simulink model "towing_project"  (Simulink 10.1)
settings: Solver=ode4  StartTime=0.0  StopTime=1000  FixedStep=1  RelTol=1e-3  EnableMultiTasking=on
PreLoadFcn:
  | load('Initialization_data.mat');
values from neighbouring files (symbols this model uses):
  D1 = [MM(1,1)/100, 0, 0; 0, MM(2,2)/40, 0; 0, 0, MM(3,3)/20]    [initail_data.m]
  M1 = diag([6.25e5, 6.25e5, 6.25e5*7.5^2])    [initail_data.m]
  Ma1 = [7.58e4, 0, 0; 0, 3.69e5 -1.4e5; 0, -1.4e5, 8.77e6]    [initail_data.m]
  p00 = [0, 0, 0]'    [initail_data.m]
  p10 = [394, 237, 31]'    [initail_data.m]
  p20 = [394, -237, -31]'    [initail_data.m]
undefined symbols (not defined in the file or in its folder): D, M, Ma, magnitude
libraries: simulink x6, simulink_extras x2
settings Model: Creator=Lither  LastModifiedBy=Administrator
settings DataIOCC: LimitDataPoints=on
settings OptimizationCC: ExpressionDepthLimit=2147483647
settings DebuggingCC: FcnCallInpInsideContextMsg=warning  StateNameClashWarn=warning
settings ConfigComp: CovSFcnEnable=off

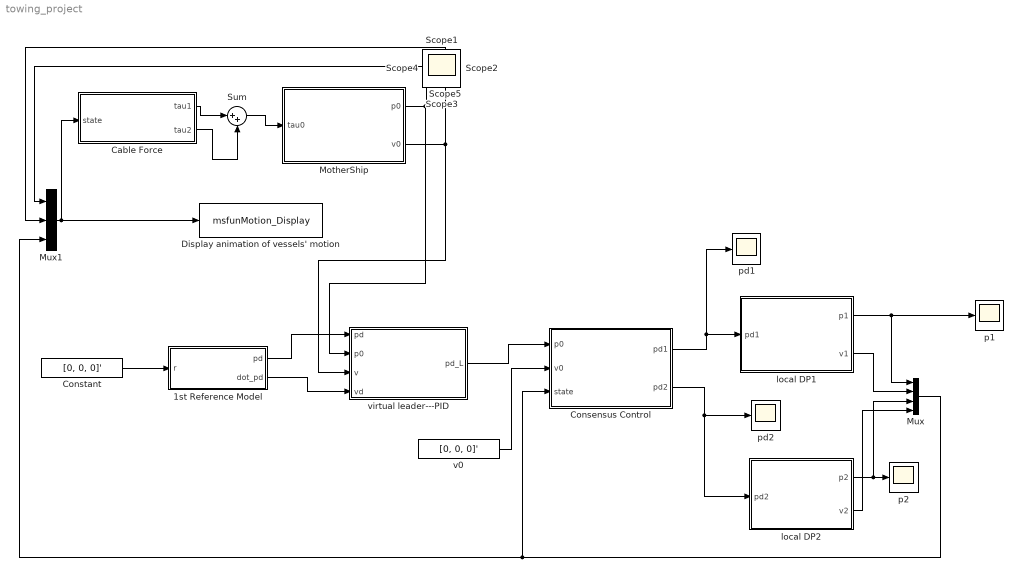
== system towing_project ==
  1st Reference Model : Subsystem  mask{T=200}
      mask prompts: T "Time constant of reference model"
  Cable Force : MATLAB Function  TreatAsAtomicUnit=on
  Consensus Control : MATLAB Function  TreatAsAtomicUnit=on
  Constant : Constant  Value=[0, 0, 0]'
  Display animation of vessels' motion : M-S-Function  FunctionName=msfunMotion_Display  Parameters=p00, p10, p20
  MotherShip : Subsystem  mask{wv=on}
      mask prompts: wv "Display animation of the vessel's motion"
  Mux : Mux
  Mux1 : Mux  Inputs=3
  Sum : Sum  Inputs=|++
  local DP1 : Subsystem
  local DP2 : Subsystem
  p1 : Scope
  p2 : Scope
  pd1 : Scope
  pd2 : Scope
  v0 : Constant  Value=[0, 0, 0]'
  virtual leader---PID : Subsystem  mask{Kp_L=diag([1, 1, 1]), Kd_L=diag([1, 1, 1])*0.1, Ki_L=diag([1, 1, 1])*0.01}
      mask prompts: Kp_L "比例增益：Kp_L"; Kd_L "微分增益：Kd_L"; Ki_L "积分增益：Ki_L"
  Scope{,1..5} (6 alike) : Scope
  wires:
  Consensus Control/1(pd1) -> pd1/1, local DP1/1(pd1)
  local DP1/1(p1) -> p1/1, Mux/1
  local DP1/2(v1) -> Mux/2
  local DP2/1(p2) -> Mux/3, p2/1
  local DP2/2(v2) -> Mux/4
  Mux/1 -> Consensus Control/3(state), Mux1/3
  Consensus Control/2(pd2) -> local DP2/1(pd2), pd2/1
  Mux1/1 -> Display animation of vessels' motion/1, Cable Force/1(state)
  Constant/1 -> 1st Reference Model/1(r)
  MotherShip/1(p0) -> virtual leader---PID/2(p0), Mux1/1
  MotherShip/2(v0) -> Mux1/2, virtual leader---PID/3(v)
  Sum/1 -> MotherShip/1(tau0)
  1st Reference Model/1(pd) -> virtual leader---PID/1(pd)
  1st Reference Model/2(dot_pd) -> virtual leader---PID/4(vd)
  virtual leader---PID/1(pd_L) -> Consensus Control/1(p0)
  v0/1 -> Consensus Control/2(v0)
  Cable Force/1(tau1) -> Sum/1
  Cable Force/2(tau2) -> Sum/2

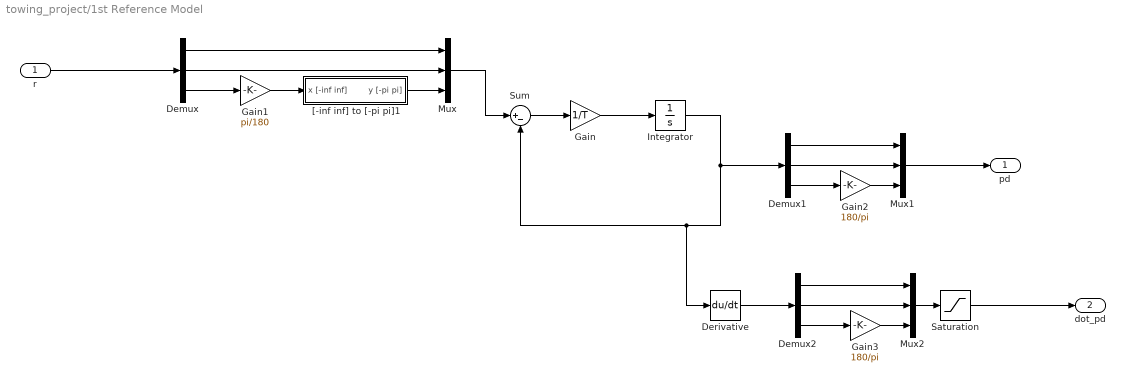
== system towing_project/1st Reference Model ==
  r : Inport
  Demux : Demux  Outputs=3
  Demux1 : Demux  Outputs=3
  Demux2 : Demux  Outputs=3
  Derivative : Derivative
  Gain : Gain  Gain=1/T
  Gain1 : Gain  Gain=pi/180
  Gain2 : Gain  Gain=180/pi
  Gain3 : Gain  Gain=180/pi
  Integrator : Integrator  InitialCondition=p00
  Mux : Mux  Inputs=3
  Mux1 : Mux  Inputs=3
  Mux2 : Mux  Inputs=3
  Saturation : Saturate  UpperLimit=10  LowerLimit=-10
  Sum : Sum  Inputs=|+-
  "[-inf inf] to [-pi pi]1" : Subsystem
  pd : Outport
  dot_pd : Outport  Port=2
  wires:
  Integrator/1 -> Derivative/1, Sum/2, Demux1/1
  Sum/1 -> Gain/1
  Gain/1 -> Integrator/1
  Saturation/1 -> dot_pd/1
  r/1 -> Demux/1
  Demux/3 -> Gain1/1
  Demux/2 -> Mux/2
  Demux/1 -> Mux/1
  Mux/1 -> Sum/1
  Demux1/3 -> Gain2/1
  Gain2/1 -> Mux1/3
  Demux1/2 -> Mux1/2
  Demux1/1 -> Mux1/1
  Mux1/1 -> pd/1
  Demux2/3 -> Gain3/1
  Demux2/2 -> Mux2/2
  Demux2/1 -> Mux2/1
  Gain3/1 -> Mux2/3
  Derivative/1 -> Demux2/1
  Mux2/1 -> Saturation/1
  Gain1/1 -> "[-inf inf] to [-pi pi]1"/1(x [-inf inf])
  "[-inf inf] to [-pi pi]1"/1(y [-pi pi]) -> Mux/3

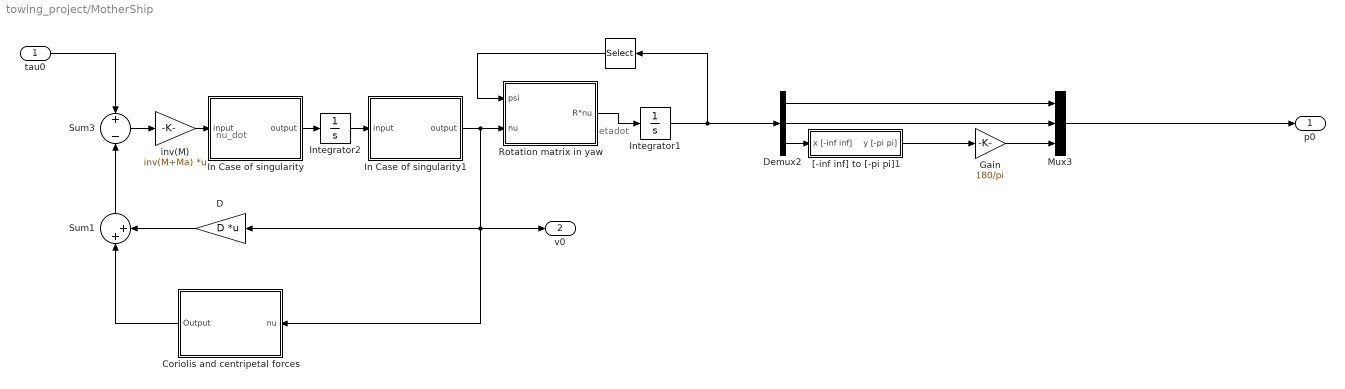
== system towing_project/MotherShip ==
  note: nu_dot
  note: etadot
  tau0 : Inport
  " " : Selector  InputPortWidth=3  IndexOptions=Index vector (dialog)  Indices=[3]  OutputSizes=1
  Coriolis and centripetal forces : Subsystem
  D : Gain  Gain=D  Multiplication=Matrix(K*u)  SaturateOnIntegerOverflow=on  OutDataTypeStr=Inherit: Same as input  ParamDataTypeStr=Inherit: Same as input
  Demux2 : Demux  Outputs=3
  Gain : Gain  Gain=180/pi
  In Case of singularity : Subsystem
  In Case of singularity1 : Subsystem
  Integrator1 : Integrator  InitialCondition=[p00(1), p00(2), p00(3)/180*pi]'
  Integrator2 : Integrator
  Mux3 : Mux  Inputs=3
  Rotation matrix in yaw : Subsystem
  Sum1 : Sum  Inputs=|++  InputSameDT=on  SaturateOnIntegerOverflow=on  OutDataTypeStr=Inherit: Same as first input
  Sum3 : Sum  Inputs=+-  InputSameDT=on  SaturateOnIntegerOverflow=on  OutDataTypeStr=Inherit: Same as first input
  "[-inf inf] to [-pi pi]1" : Subsystem
  inv(M) : Gain  Gain=inv(M+Ma)  Multiplication=Matrix(K*u)  SaturateOnIntegerOverflow=on  OutDataTypeStr=Inherit: Same as input  ParamDataTypeStr=Inherit: Same as input
  p0 : Outport
  v0 : Outport  Port=2
  wires:
  Sum3/1 -> inv(M)/1
  inv(M)/1 -> In Case of singularity/1(input)
  Rotation matrix in yaw/1(R*nu) -> Integrator1/1
  Integrator1/1 -> Demux2/1, " "/1
  " "/1 -> Rotation matrix in yaw/1(psi)
  tau0/1 -> Sum3/1
  Integrator2/1 -> In Case of singularity1/1(input)
  In Case of singularity/1(output) -> Integrator2/1
  In Case of singularity1/1(output) -> Rotation matrix in yaw/2(nu), D/1, Coriolis and centripetal forces/1(nu), v0/1
  D/1 -> Sum1/2
  Coriolis and centripetal forces/1(Output) -> Sum1/1
  Sum1/1 -> Sum3/2
  Demux2/3 -> "[-inf inf] to [-pi pi]1"/1(x [-inf inf])
  Demux2/1 -> Mux3/1
  Demux2/2 -> Mux3/2
  Mux3/1 -> p0/1
  "[-inf inf] to [-pi pi]1"/1(y [-pi pi]) -> Gain/1
  Gain/1 -> Mux3/3

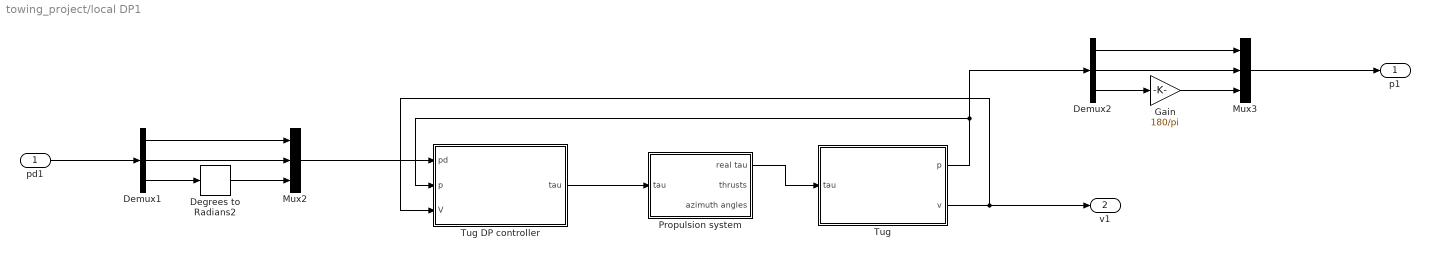
== system towing_project/local DP1 ==
  pd1 : Inport
  Degrees to Radians2 : simulink_extras/Transformations/Degrees to Radians
  Demux1 : Demux  Outputs=3
  Demux2 : Demux  Outputs=3
  Gain : Gain  Gain=180/pi
  Mux2 : Mux  Inputs=3
  Mux3 : Mux  Inputs=3
  Propulsion system : Subsystem  mask{f0=[1;1;1], a0=[50;60;70], u0=[1; 1; 1], wa=on}
      mask prompts: f0 "Initial values of thrusts"; a0 "Initial values of azimuth angles"; u0 "Thruster utilization"; wa "Show animation of thrust and azimuth angle"
  Tug : Subsystem  mask{wv=on}
      mask prompts: wv "Display animation of the vessel's motion"
  Tug DP controller : Subsystem  mask(Nonlinear DP Controller){Kp=diag([0.0028, 0.004, 0.0031]), Kd=diag([0.0573, 0.0716, 0.025]), Ki=diag([0.0028, 0.004, 0.0031])*0.01, WFF_gain=0}
      mask prompts: Kp "Proportional Gain Matrix: Kp"; Kd "Derivative Gain Matrix: Kd"; Ki "Integral Gain Matrix: Ki"; WFF_gain "Wave feedforward Gain"
      mask help: PID controller for Set-Point Reulation in Surge, Sway and Yaw
      mask Help:
      | The nonlinear  PID controller uses the rotation matrix in yaw for proper scaling of the surge, sway and yaw gains as a function of the yaw angle.
      | INPUTS: (1) eta_ref, (2) eta, (3) nu. OUPUTS: (1) tau.
      mask Display: disp('PID controller')
  p1 : Outport
  v1 : Outport  Port=2
  wires:
  Tug/2(v) -> v1/1, Tug DP controller/3(V)
  Tug DP controller/1(tau) -> Propulsion system/1(tau)
  Demux1/2 -> Mux2/2
  Mux2/1 -> Tug DP controller/1(pd)
  Demux1/1 -> Mux2/1
  Degrees to Radians2/1 -> Mux2/3
  Demux1/3 -> Degrees to Radians2/1
  pd1/1 -> Demux1/1
  Propulsion system/1(real tau) -> Tug/1(tau)
  Demux2/2 -> Mux3/2
  Tug/1(p) -> Demux2/1, Tug DP controller/2(p)
  Mux3/1 -> p1/1
  Demux2/3 -> Gain/1
  Gain/1 -> Mux3/3
  Demux2/1 -> Mux3/1

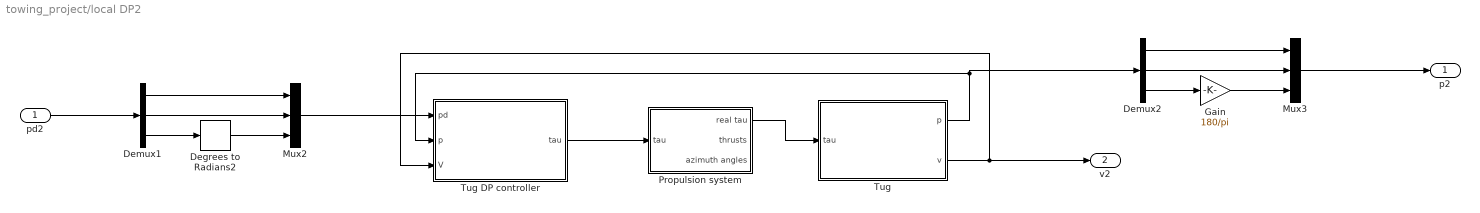
== system towing_project/local DP2 ==
  pd2 : Inport
  Degrees to Radians2 : simulink_extras/Transformations/Degrees to Radians
  Demux1 : Demux  Outputs=3
  Demux2 : Demux  Outputs=3
  Gain : Gain  Gain=180/pi
  Mux2 : Mux  Inputs=3
  Mux3 : Mux  Inputs=3
  Propulsion system : Subsystem  mask{f0=[1;1;1], a0=[50;60;70], u0=[1; 1; 1], wa=on}
      mask prompts: f0 "Initial values of thrusts"; a0 "Initial values of azimuth angles"; u0 "Thruster utilization"; wa "Show animation of thrust and azimuth angle"
  Tug : Subsystem  mask{wv=on}
      mask prompts: wv "Display animation of the vessel's motion"
  Tug DP controller : Subsystem  mask(Nonlinear DP Controller){Kp=diag([0.0028, 0.004, 0.0031]), Kd=diag([0.0573, 0.0716, 0.025]), Ki=diag([0.0028, 0.004, 0.0031])*0.01, WFF_gain=0}
      mask prompts: Kp "Proportional Gain Matrix: Kp"; Kd "Derivative Gain Matrix: Kd"; Ki "Integral Gain Matrix: Ki"; WFF_gain "Wave feedforward Gain"
      mask help: PID controller for Set-Point Reulation in Surge, Sway and Yaw
      mask Help:
      | The nonlinear  PID controller uses the rotation matrix in yaw for proper scaling of the surge, sway and yaw gains as a function of the yaw angle.
      | INPUTS: (1) eta_ref, (2) eta, (3) nu. OUPUTS: (1) tau.
      mask Display: disp('PID controller')
  p2 : Outport
  v2 : Outport  Port=2
  wires:
  Tug/2(v) -> v2/1, Tug DP controller/3(V)
  Tug DP controller/1(tau) -> Propulsion system/1(tau)
  Demux1/2 -> Mux2/2
  Mux2/1 -> Tug DP controller/1(pd)
  Demux1/1 -> Mux2/1
  Degrees to Radians2/1 -> Mux2/3
  Demux1/3 -> Degrees to Radians2/1
  pd2/1 -> Demux1/1
  Propulsion system/1(real tau) -> Tug/1(tau)
  Mux3/1 -> p2/1
  Tug/1(p) -> Demux2/1, Tug DP controller/2(p)
  Demux2/3 -> Gain/1
  Demux2/2 -> Mux3/2
  Gain/1 -> Mux3/3
  Demux2/1 -> Mux3/1

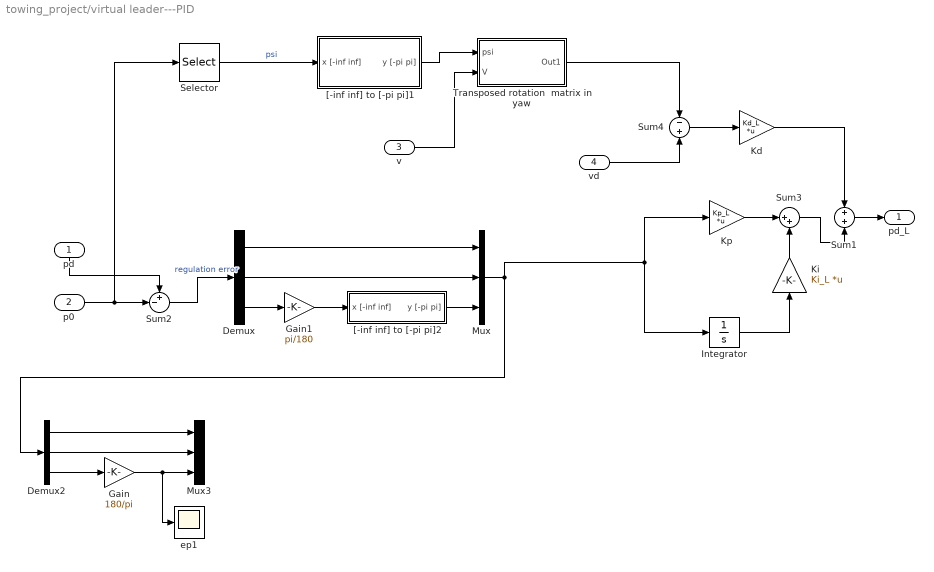
== system towing_project/virtual leader---PID ==
  pd : Inport
  p0 : Inport  Port=2
  v : Inport  Port=3
  vd : Inport  Port=4
  Demux : Demux  Outputs=3
  Demux2 : Demux  Outputs=3
  Gain : Gain  Gain=180/pi
  Gain1 : Gain  Gain=pi/180
  Integrator : Integrator
  Kd : Gain  Gain=Kd_L  Multiplication=Matrix(K*u)  SaturateOnIntegerOverflow=on  OutDataTypeStr=Inherit: Same as input  ParamDataTypeStr=Inherit: Same as input
  Ki : Gain  Gain=Ki_L  Multiplication=Matrix(K*u)  SaturateOnIntegerOverflow=on  OutDataTypeStr=Inherit: Same as input  ParamDataTypeStr=Inherit: Same as input
  Kp : Gain  Gain=Kp_L  Multiplication=Matrix(K*u)  SaturateOnIntegerOverflow=on  OutDataTypeStr=Inherit: Same as input  ParamDataTypeStr=Inherit: Same as input
  Mux : Mux  Inputs=3
  Mux3 : Mux  Inputs=3
  Selector : Selector  InputPortWidth=3  IndexOptions=Index vector (dialog)  Indices=[ 3]  OutputSizes=1
  Sum1 : Sum  InputSameDT=on  SaturateOnIntegerOverflow=on  OutDataTypeStr=Inherit: Same as first input
  Sum2 : Sum  Inputs=+-|  InputSameDT=on  SaturateOnIntegerOverflow=on  OutDataTypeStr=Inherit: Same as first input
  Sum3 : Sum  Inputs=|++  InputSameDT=on  SaturateOnIntegerOverflow=on  OutDataTypeStr=Inherit: Same as first input
  Sum4 : Sum  Inputs=-+  InputSameDT=on  SaturateOnIntegerOverflow=on  OutDataTypeStr=Inherit: Same as first input
  Transposed rotation  matrix in yaw : Subsystem
  "[-inf inf] to [-pi pi]1" : Subsystem
  "[-inf inf] to [-pi pi]2" : Subsystem
  ep1 : Scope
  pd_L : Outport  InitialOutput=0
  wires:
  Gain/1 -> ep1/1, Mux3/3
  Demux2/1 -> Mux3/1
  Kp/1 -> Sum3/1
  "[-inf inf] to [-pi pi]1"/1(y [-pi pi]) -> Transposed rotation  matrix in yaw/1(psi)
  Demux2/3 -> Gain/1
  Demux2/2 -> Mux3/2
  Integrator/1 -> Ki/1
  Sum1/1 -> pd_L/1
  p0/1 -> Sum2/2, Selector/1
  Sum2/1 -> Demux/1  "regulation error"
  pd/1 -> Sum2/1
  Mux/1 -> Demux2/1, Kp/1, Integrator/1
  Demux/1 -> Mux/1
  Selector/1 -> "[-inf inf] to [-pi pi]1"/1(x [-inf inf])  "psi"
  Ki/1 -> Sum3/2
  Demux/2 -> Mux/2
  "[-inf inf] to [-pi pi]2"/1(y [-pi pi]) -> Mux/3
  Demux/3 -> Gain1/1
  Gain1/1 -> "[-inf inf] to [-pi pi]2"/1(x [-inf inf])
  v/1 -> Transposed rotation  matrix in yaw/2(V)
  Sum4/1 -> Kd/1
  Kd/1 -> Sum1/1
  Sum3/1 -> Sum1/2
  Transposed rotation  matrix in yaw/1(Out1) -> Sum4/1
  vd/1 -> Sum4/2

== system towing_project/1st Reference Model/[-inf inf] to [-pi pi]1 ==
  note: x
  note: r
  x [-inf inf] : Inport
  Constant : Constant  Value=2*pi
  Gain : Gain  Gain=pi  SaturateOnIntegerOverflow=on  OutDataTypeStr=Inherit: Same as input  ParamDataTypeStr=Inherit: Same as input
  Math Function : Math  Operator=rem  SignedPower=on  SaturateOnIntegerOverflow=on
  Saturation : Saturate  UpperLimit=1e10  LowerLimit=-1e10
  Sign : Signum
  Sum : Sum  Inputs=|+-  SaturateOnIntegerOverflow=on
  Sum1 : Sum  Inputs=|++  SaturateOnIntegerOverflow=on
  y [-pi pi] : Outport
  wires:
  x [-inf inf]/1 -> Saturation/1
  Sign/1 -> Gain/1
  Gain/1 -> Sum/2, Sum1/2
  Sum1/1 -> Math Function/1
  Constant/1 -> Math Function/2
  Math Function/1 -> Sum/1
  Sum/1 -> y [-pi pi]/1
  Saturation/1 -> Sum1/1, Sign/1

== system towing_project/MotherShip/Coriolis and centripetal forces ==
  nu : Inport
  Mux : Mux  Inputs=3
  Selector1 : Selector  InputPortWidth=3  IndexOptions=Index vector (dialog)  Indices=[1 ]  OutputSizes=1
  Selector2 : Selector  InputPortWidth=3  IndexOptions=Index vector (dialog)  Indices=[2]  OutputSizes=1
  Selector3 : Selector  InputPortWidth=3  IndexOptions=Index vector (dialog)  Indices=[3]  OutputSizes=1
  Subsystem : Subsystem
  Subsystem1 : Subsystem
  Subsystem2 : Subsystem
  Output : Outport
  wires:
  nu/1 -> Selector1/1, Selector2/1, Selector3/1
  Selector2/1 -> Subsystem/1(v), Subsystem2/2(v)  "v"
  Selector3/1 -> Subsystem/2(r), Subsystem1/2(r), Subsystem2/3(r)  "r"
  Selector1/1 -> Subsystem1/1(u), Subsystem2/1(u)  "u"
  Subsystem/1(x direction) -> Mux/1
  Subsystem1/1(y direction) -> Mux/2
  Subsystem2/1(yaw direction) -> Mux/3
  Mux/1 -> Output/1

== system towing_project/MotherShip/In Case of singularity ==
  input : Inport
  Compare To Constant : simulink/Logic and Bit Operations/Compare To Constant  relop=>=  const=1e8  OutDataTypeStr=boolean
  Stop Simulation : Stop
  output : Outport
  wires:
  input/1 -> output/1, Compare To Constant/1
  Compare To Constant/1 -> Stop Simulation/1

== system towing_project/MotherShip/In Case of singularity1 ==
  input : Inport
  Compare To Constant : simulink/Logic and Bit Operations/Compare To Constant  relop=>=  const=1e10  OutDataTypeStr=boolean
  Stop Simulation : Stop
  output : Outport
  wires:
  input/1 -> output/1, Compare To Constant/1
  Compare To Constant/1 -> Stop Simulation/1

== system towing_project/MotherShip/Rotation matrix in yaw ==
  psi : Inport
  nu : Inport  Port=2
  Fcn : Fcn  Expr=cos(u(1))*u(2)-sin(u(1))*u(3)
  Fcn1 : Fcn  Expr=sin(u(1))*u(2)+cos(u(1))*u(3)
  Fcn2 : Fcn  Expr=u(4)
  Mux : Mux  Inputs=2
  Mux1 : Mux  Inputs=3
  R*nu : Outport
  wires:
  Mux1/1 -> R*nu/1  "eta_dot"
  Mux/1 -> Fcn/1, Fcn1/1, Fcn2/1
  psi/1 -> Mux/1
  nu/1 -> Mux/2
  Fcn1/1 -> Mux1/2  "y_dot"
  Fcn/1 -> Mux1/1  "x_dot"
  Fcn2/1 -> Mux1/3  "psi_dot"

== system towing_project/MotherShip/[-inf inf] to [-pi pi]1 ==
  note: x
  note: r
  x [-inf inf] : Inport
  Constant : Constant  Value=2*pi
  Gain : Gain  Gain=pi  SaturateOnIntegerOverflow=on  OutDataTypeStr=Inherit: Same as input  ParamDataTypeStr=Inherit: Same as input
  Math Function : Math  Operator=rem  SignedPower=on  SaturateOnIntegerOverflow=on
  Saturation : Saturate  UpperLimit=1e10  LowerLimit=-1e10
  Sign : Signum
  Sum : Sum  Inputs=|+-  SaturateOnIntegerOverflow=on
  Sum1 : Sum  Inputs=|++  SaturateOnIntegerOverflow=on
  y [-pi pi] : Outport
  wires:
  x [-inf inf]/1 -> Saturation/1
  Sign/1 -> Gain/1
  Gain/1 -> Sum/2, Sum1/2
  Sum1/1 -> Math Function/1
  Constant/1 -> Math Function/2
  Math Function/1 -> Sum/1
  Sum/1 -> y [-pi pi]/1
  Saturation/1 -> Sum1/1, Sign/1

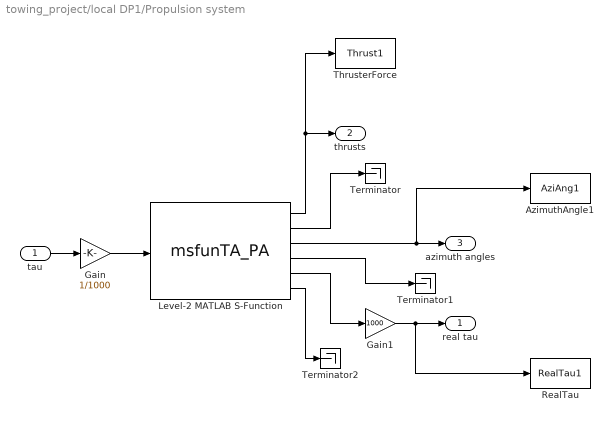
== system towing_project/local DP1/Propulsion system ==
  tau : Inport
  AzimuthAngle1 : ToWorkspace  VariableName=AziAng1  SampleTime=-1
  Gain : Gain  Gain=1/1000
  Gain1 : Gain  Gain=1000
  Level-2 MATLAB S-Function : M-S-Function  FunctionName=msfunTA_PA  Parameters=f0,a0,wa
  RealTau : ToWorkspace  VariableName=RealTau1  SampleTime=-1
  Terminator : Terminator
  Terminator1 : Terminator
  Terminator2 : Terminator
  ThrusterForce : ToWorkspace  VariableName=Thrust1  SampleTime=-1
  real tau : Outport
  thrusts : Outport  Port=2
  azimuth angles : Outport  Port=3
  wires:
  tau/1 -> Gain/1
  Level-2 MATLAB S-Function/2 -> Terminator/1
  Level-2 MATLAB S-Function/3 -> AzimuthAngle1/1, azimuth angles/1
  Level-2 MATLAB S-Function/4 -> Terminator1/1
  Level-2 MATLAB S-Function/5 -> Gain1/1
  Level-2 MATLAB S-Function/6 -> Terminator2/1
  Level-2 MATLAB S-Function/1 -> ThrusterForce/1, thrusts/1
  Gain/1 -> Level-2 MATLAB S-Function/1
  Gain1/1 -> RealTau/1, real tau/1

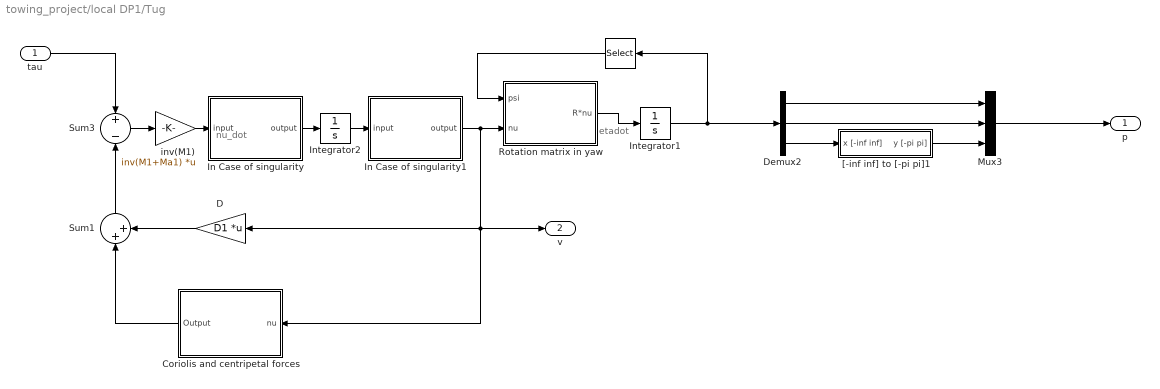
== system towing_project/local DP1/Tug ==
  note: nu_dot
  note: etadot
  tau : Inport
  " " : Selector  InputPortWidth=3  IndexOptions=Index vector (dialog)  Indices=[3]  OutputSizes=1
  Coriolis and centripetal forces : Subsystem
  D : Gain  Gain=D1  Multiplication=Matrix(K*u)  SaturateOnIntegerOverflow=on  OutDataTypeStr=Inherit: Same as input  ParamDataTypeStr=Inherit: Same as input
  Demux2 : Demux  Outputs=3
  In Case of singularity : Subsystem
  In Case of singularity1 : Subsystem
  Integrator1 : Integrator  InitialCondition=[p10(1), p10(2), p10(3)/180*pi]'
  Integrator2 : Integrator
  Mux3 : Mux  Inputs=3
  Rotation matrix in yaw : Subsystem
  Sum1 : Sum  Inputs=|++  InputSameDT=on  SaturateOnIntegerOverflow=on  OutDataTypeStr=Inherit: Same as first input
  Sum3 : Sum  Inputs=+-  InputSameDT=on  SaturateOnIntegerOverflow=on  OutDataTypeStr=Inherit: Same as first input
  "[-inf inf] to [-pi pi]1" : Subsystem
  inv(M1) : Gain  Gain=inv(M1+Ma1)  Multiplication=Matrix(K*u)  SaturateOnIntegerOverflow=on  OutDataTypeStr=Inherit: Same as input  ParamDataTypeStr=Inherit: Same as input
  p : Outport
  v : Outport  Port=2
  wires:
  Sum3/1 -> inv(M1)/1
  inv(M1)/1 -> In Case of singularity/1(input)
  Rotation matrix in yaw/1(R*nu) -> Integrator1/1
  Integrator1/1 -> Demux2/1, " "/1
  " "/1 -> Rotation matrix in yaw/1(psi)
  tau/1 -> Sum3/1
  Integrator2/1 -> In Case of singularity1/1(input)
  In Case of singularity/1(output) -> Integrator2/1
  In Case of singularity1/1(output) -> Rotation matrix in yaw/2(nu), D/1, Coriolis and centripetal forces/1(nu), v/1
  D/1 -> Sum1/2
  Coriolis and centripetal forces/1(Output) -> Sum1/1
  Sum1/1 -> Sum3/2
  Demux2/3 -> "[-inf inf] to [-pi pi]1"/1(x [-inf inf])
  Demux2/1 -> Mux3/1
  Demux2/2 -> Mux3/2
  "[-inf inf] to [-pi pi]1"/1(y [-pi pi]) -> Mux3/3
  Mux3/1 -> p/1

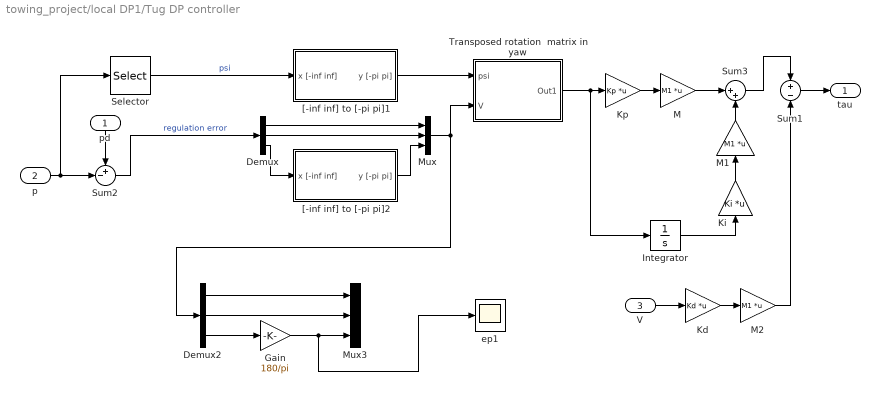
== system towing_project/local DP1/Tug DP controller ==
  pd : Inport
  p : Inport  Port=2
  V : Inport  Port=3
  Demux : Demux  Outputs=3
  Demux2 : Demux  Outputs=3
  Gain : Gain  Gain=180/pi
  Integrator : Integrator
  Kd : Gain  Gain=Kd  Multiplication=Matrix(K*u)  SaturateOnIntegerOverflow=on  OutDataTypeStr=Inherit: Same as input  ParamDataTypeStr=Inherit: Same as input
  Ki : Gain  Gain=Ki  Multiplication=Matrix(K*u)  SaturateOnIntegerOverflow=on  OutDataTypeStr=Inherit: Same as input  ParamDataTypeStr=Inherit: Same as input
  Kp : Gain  Gain=Kp  Multiplication=Matrix(K*u)  SaturateOnIntegerOverflow=on  OutDataTypeStr=Inherit: Same as input  ParamDataTypeStr=Inherit: Same as input
  M : Gain  Gain=M1  Multiplication=Matrix(K*u)  SaturateOnIntegerOverflow=on  OutDataTypeStr=Inherit: Same as input  ParamDataTypeStr=Inherit: Same as input
  M1 : Gain  Gain=M1  Multiplication=Matrix(K*u)  SaturateOnIntegerOverflow=on  OutDataTypeStr=Inherit: Same as input  ParamDataTypeStr=Inherit: Same as input
  M2 : Gain  Gain=M1  Multiplication=Matrix(K*u)  SaturateOnIntegerOverflow=on  OutDataTypeStr=Inherit: Same as input  ParamDataTypeStr=Inherit: Same as input
  Mux : Mux  Inputs=3
  Mux3 : Mux  Inputs=3
  Selector : Selector  InputPortWidth=3  IndexOptions=Index vector (dialog)  Indices=[ 3]  OutputSizes=1
  Sum1 : Sum  Inputs=+-  InputSameDT=on  SaturateOnIntegerOverflow=on  OutDataTypeStr=Inherit: Same as first input
  Sum2 : Sum  Inputs=+-|  InputSameDT=on  SaturateOnIntegerOverflow=on  OutDataTypeStr=Inherit: Same as first input
  Sum3 : Sum  Inputs=|++  InputSameDT=on  SaturateOnIntegerOverflow=on  OutDataTypeStr=Inherit: Same as first input
  Transposed rotation  matrix in yaw : Subsystem
  "[-inf inf] to [-pi pi]1" : Subsystem
  "[-inf inf] to [-pi pi]2" : Subsystem
  ep1 : Scope
  tau : Outport  InitialOutput=0
  wires:
  "[-inf inf] to [-pi pi]1"/1(y [-pi pi]) -> Transposed rotation  matrix in yaw/1(psi)
  Selector/1 -> "[-inf inf] to [-pi pi]1"/1(x [-inf inf])  "psi"
  Mux/1 -> Demux2/1, Transposed rotation  matrix in yaw/2(V)
  Demux/1 -> Mux/1
  Demux/2 -> Mux/2
  "[-inf inf] to [-pi pi]2"/1(y [-pi pi]) -> Mux/3
  Sum2/1 -> Demux/1  "regulation error"
  Demux/3 -> "[-inf inf] to [-pi pi]2"/1(x [-inf inf])
  pd/1 -> Sum2/1
  Sum1/1 -> tau/1
  p/1 -> Sum2/2, Selector/1
  V/1 -> Kd/1
  Integrator/1 -> Ki/1
  Kp/1 -> M/1
  Ki/1 -> M1/1
  Transposed rotation  matrix in yaw/1(Out1) -> Kp/1, Integrator/1
  Kd/1 -> M2/1
  M/1 -> Sum3/1
  M1/1 -> Sum3/2
  Sum3/1 -> Sum1/1
  M2/1 -> Sum1/2
  Demux2/3 -> Gain/1
  Demux2/1 -> Mux3/1
  Demux2/2 -> Mux3/2
  Gain/1 -> ep1/1, Mux3/3

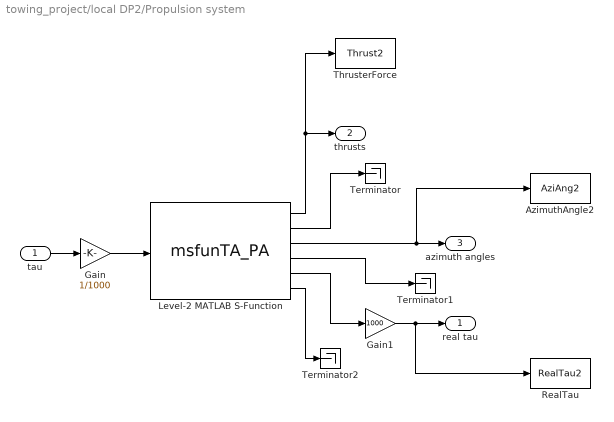
== system towing_project/local DP2/Propulsion system ==
  tau : Inport
  AzimuthAngle2 : ToWorkspace  VariableName=AziAng2  SampleTime=-1
  Gain : Gain  Gain=1/1000
  Gain1 : Gain  Gain=1000
  Level-2 MATLAB S-Function : M-S-Function  FunctionName=msfunTA_PA  Parameters=f0,a0,wa
  RealTau : ToWorkspace  VariableName=RealTau2  SampleTime=-1
  Terminator : Terminator
  Terminator1 : Terminator
  Terminator2 : Terminator
  ThrusterForce : ToWorkspace  VariableName=Thrust2  SampleTime=-1
  real tau : Outport
  thrusts : Outport  Port=2
  azimuth angles : Outport  Port=3
  wires:
  tau/1 -> Gain/1
  Level-2 MATLAB S-Function/2 -> Terminator/1
  Level-2 MATLAB S-Function/3 -> AzimuthAngle2/1, azimuth angles/1
  Level-2 MATLAB S-Function/4 -> Terminator1/1
  Level-2 MATLAB S-Function/5 -> Gain1/1
  Level-2 MATLAB S-Function/6 -> Terminator2/1
  Level-2 MATLAB S-Function/1 -> ThrusterForce/1, thrusts/1
  Gain/1 -> Level-2 MATLAB S-Function/1
  Gain1/1 -> RealTau/1, real tau/1

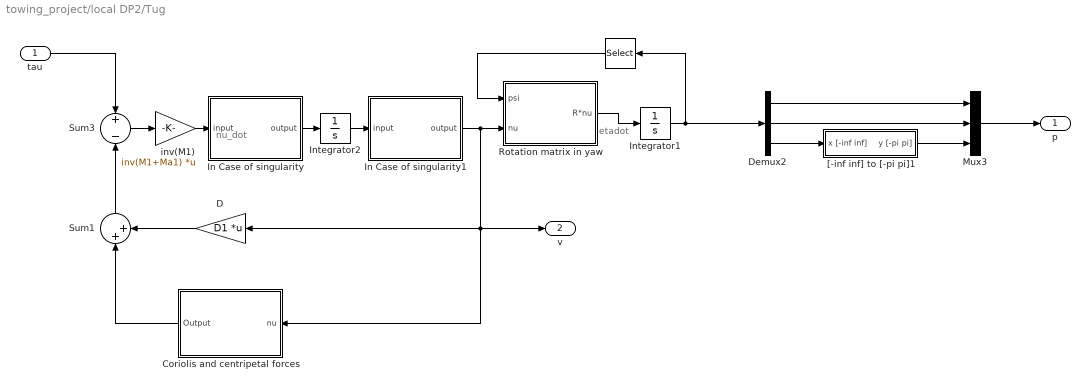
== system towing_project/local DP2/Tug ==
  note: nu_dot
  note: etadot
  tau : Inport
  " " : Selector  InputPortWidth=3  IndexOptions=Index vector (dialog)  Indices=[3]  OutputSizes=1
  Coriolis and centripetal forces : Subsystem
  D : Gain  Gain=D1  Multiplication=Matrix(K*u)  SaturateOnIntegerOverflow=on  OutDataTypeStr=Inherit: Same as input  ParamDataTypeStr=Inherit: Same as input
  Demux2 : Demux  Outputs=3
  In Case of singularity : Subsystem
  In Case of singularity1 : Subsystem
  Integrator1 : Integrator  InitialCondition=[p20(1), p20(2), p20(3)/180*pi]'
  Integrator2 : Integrator
  Mux3 : Mux  Inputs=3
  Rotation matrix in yaw : Subsystem
  Sum1 : Sum  Inputs=|++  InputSameDT=on  SaturateOnIntegerOverflow=on  OutDataTypeStr=Inherit: Same as first input
  Sum3 : Sum  Inputs=+-  InputSameDT=on  SaturateOnIntegerOverflow=on  OutDataTypeStr=Inherit: Same as first input
  "[-inf inf] to [-pi pi]1" : Subsystem
  inv(M1) : Gain  Gain=inv(M1+Ma1)  Multiplication=Matrix(K*u)  SaturateOnIntegerOverflow=on  OutDataTypeStr=Inherit: Same as input  ParamDataTypeStr=Inherit: Same as input
  p : Outport
  v : Outport  Port=2
  wires:
  Sum3/1 -> inv(M1)/1
  inv(M1)/1 -> In Case of singularity/1(input)
  Rotation matrix in yaw/1(R*nu) -> Integrator1/1
  " "/1 -> Rotation matrix in yaw/1(psi)
  tau/1 -> Sum3/1
  Integrator2/1 -> In Case of singularity1/1(input)
  In Case of singularity/1(output) -> Integrator2/1
  In Case of singularity1/1(output) -> Rotation matrix in yaw/2(nu), D/1, Coriolis and centripetal forces/1(nu), v/1
  D/1 -> Sum1/2
  Coriolis and centripetal forces/1(Output) -> Sum1/1
  Sum1/1 -> Sum3/2
  Demux2/3 -> "[-inf inf] to [-pi pi]1"/1(x [-inf inf])
  Integrator1/1 -> " "/1, Demux2/1
  "[-inf inf] to [-pi pi]1"/1(y [-pi pi]) -> Mux3/3
  Demux2/2 -> Mux3/2
  Demux2/1 -> Mux3/1
  Mux3/1 -> p/1

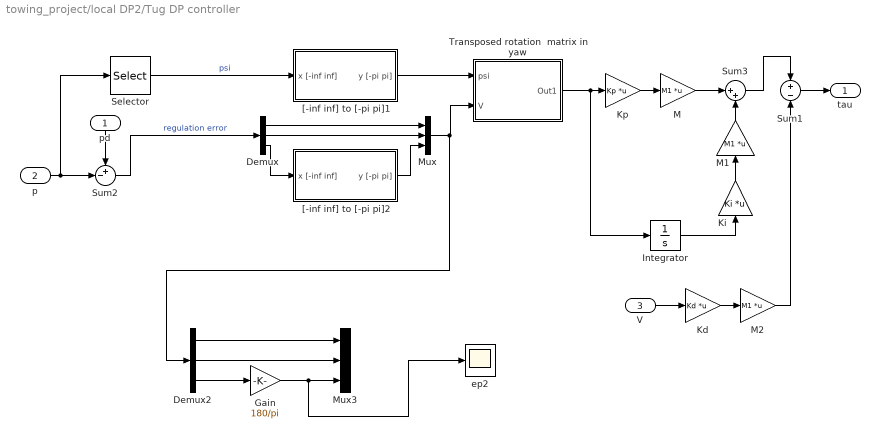
== system towing_project/local DP2/Tug DP controller ==
  pd : Inport
  p : Inport  Port=2
  V : Inport  Port=3
  Demux : Demux  Outputs=3
  Demux2 : Demux  Outputs=3
  Gain : Gain  Gain=180/pi
  Integrator : Integrator
  Kd : Gain  Gain=Kd  Multiplication=Matrix(K*u)  SaturateOnIntegerOverflow=on  OutDataTypeStr=Inherit: Same as input  ParamDataTypeStr=Inherit: Same as input
  Ki : Gain  Gain=Ki  Multiplication=Matrix(K*u)  SaturateOnIntegerOverflow=on  OutDataTypeStr=Inherit: Same as input  ParamDataTypeStr=Inherit: Same as input
  Kp : Gain  Gain=Kp  Multiplication=Matrix(K*u)  SaturateOnIntegerOverflow=on  OutDataTypeStr=Inherit: Same as input  ParamDataTypeStr=Inherit: Same as input
  M : Gain  Gain=M1  Multiplication=Matrix(K*u)  SaturateOnIntegerOverflow=on  OutDataTypeStr=Inherit: Same as input  ParamDataTypeStr=Inherit: Same as input
  M1 : Gain  Gain=M1  Multiplication=Matrix(K*u)  SaturateOnIntegerOverflow=on  OutDataTypeStr=Inherit: Same as input  ParamDataTypeStr=Inherit: Same as input
  M2 : Gain  Gain=M1  Multiplication=Matrix(K*u)  SaturateOnIntegerOverflow=on  OutDataTypeStr=Inherit: Same as input  ParamDataTypeStr=Inherit: Same as input
  Mux : Mux  Inputs=3
  Mux3 : Mux  Inputs=3
  Selector : Selector  InputPortWidth=3  IndexOptions=Index vector (dialog)  Indices=[ 3]  OutputSizes=1
  Sum1 : Sum  Inputs=+-  InputSameDT=on  SaturateOnIntegerOverflow=on  OutDataTypeStr=Inherit: Same as first input
  Sum2 : Sum  Inputs=+-|  InputSameDT=on  SaturateOnIntegerOverflow=on  OutDataTypeStr=Inherit: Same as first input
  Sum3 : Sum  Inputs=|++  InputSameDT=on  SaturateOnIntegerOverflow=on  OutDataTypeStr=Inherit: Same as first input
  Transposed rotation  matrix in yaw : Subsystem
  "[-inf inf] to [-pi pi]1" : Subsystem
  "[-inf inf] to [-pi pi]2" : Subsystem
  ep2 : Scope
  tau : Outport  InitialOutput=0
  wires:
  "[-inf inf] to [-pi pi]1"/1(y [-pi pi]) -> Transposed rotation  matrix in yaw/1(psi)
  Selector/1 -> "[-inf inf] to [-pi pi]1"/1(x [-inf inf])  "psi"
  Demux/1 -> Mux/1
  Demux/2 -> Mux/2
  "[-inf inf] to [-pi pi]2"/1(y [-pi pi]) -> Mux/3
  Sum2/1 -> Demux/1  "regulation error"
  Demux/3 -> "[-inf inf] to [-pi pi]2"/1(x [-inf inf])
  pd/1 -> Sum2/1
  Sum1/1 -> tau/1
  p/1 -> Sum2/2, Selector/1
  V/1 -> Kd/1
  Integrator/1 -> Ki/1
  Kp/1 -> M/1
  Ki/1 -> M1/1
  Transposed rotation  matrix in yaw/1(Out1) -> Kp/1, Integrator/1
  Kd/1 -> M2/1
  M/1 -> Sum3/1
  M1/1 -> Sum3/2
  Sum3/1 -> Sum1/1
  M2/1 -> Sum1/2
  Gain/1 -> ep2/1, Mux3/3
  Demux2/1 -> Mux3/1
  Demux2/3 -> Gain/1
  Mux/1 -> Demux2/1, Transposed rotation  matrix in yaw/2(V)
  Demux2/2 -> Mux3/2

== system towing_project/virtual leader---PID/Transposed rotation  matrix in yaw ==
  psi : Inport
  V : Inport  Port=2
  Mux : Mux  Inputs=2
  Mux1 : Mux  Inputs=3
  Row1 : Fcn  Expr=cos(u(1))*u(2)-sin(u(1))*u(3)
  Row2 : Fcn  Expr=sin(u(1))*u(2)+cos(u(1))*u(3)
  Row3 : Fcn  Expr=u(4)
  Out1 : Outport
  wires:
  Mux/1 -> Row3/1, Row2/1, Row1/1
  Row1/1 -> Mux1/1
  Row2/1 -> Mux1/2
  Row3/1 -> Mux1/3
  Mux1/1 -> Out1/1
  psi/1 -> Mux/1
  V/1 -> Mux/2

== system towing_project/virtual leader---PID/[-inf inf] to [-pi pi]1 ==
  note: x
  note: r
  x [-inf inf] : Inport
  Constant : Constant  Value=2*pi
  Gain : Gain  Gain=pi  SaturateOnIntegerOverflow=on  OutDataTypeStr=Inherit: Same as input  ParamDataTypeStr=Inherit: Same as input
  Math Function : Math  Operator=rem  SignedPower=on  SaturateOnIntegerOverflow=on
  Saturation : Saturate  UpperLimit=1e10  LowerLimit=-1e10
  Sign : Signum
  Sum : Sum  Inputs=|+-  SaturateOnIntegerOverflow=on
  Sum1 : Sum  Inputs=|++  SaturateOnIntegerOverflow=on
  y [-pi pi] : Outport
  wires:
  x [-inf inf]/1 -> Saturation/1
  Sign/1 -> Gain/1
  Gain/1 -> Sum/2, Sum1/2
  Sum1/1 -> Math Function/1
  Constant/1 -> Math Function/2
  Math Function/1 -> Sum/1
  Sum/1 -> y [-pi pi]/1
  Saturation/1 -> Sum1/1, Sign/1

== system towing_project/virtual leader---PID/[-inf inf] to [-pi pi]2 ==
  note: r
  note: x
  x [-inf inf] : Inport
  Constant : Constant  Value=2*pi
  Gain : Gain  Gain=pi  SaturateOnIntegerOverflow=on  OutDataTypeStr=Inherit: Same as input  ParamDataTypeStr=Inherit: Same as input
  Math Function : Math  Operator=rem  SignedPower=on  SaturateOnIntegerOverflow=on
  Saturation : Saturate  UpperLimit=1e10  LowerLimit=-1e10
  Sign : Signum
  Sum : Sum  Inputs=|+-  SaturateOnIntegerOverflow=on
  Sum1 : Sum  Inputs=|++  SaturateOnIntegerOverflow=on
  y [-pi pi] : Outport
  wires:
  Saturation/1 -> Sign/1, Sum1/1
  Sum/1 -> y [-pi pi]/1
  Math Function/1 -> Sum/1
  Constant/1 -> Math Function/2
  Sum1/1 -> Math Function/1
  Gain/1 -> Sum1/2, Sum/2
  Sign/1 -> Gain/1
  x [-inf inf]/1 -> Saturation/1

== system towing_project/MotherShip/Coriolis and centripetal forces/Subsystem ==
  v : Inport
  r : Inport  Port=2
  -a22 : Gain  Gain=-M(2,2)-Ma(2,2)  Multiplication=Matrix(K*u)  SaturateOnIntegerOverflow=on  OutDataTypeStr=Inherit: Same as input  ParamDataTypeStr=Inherit: Same as input
  -a26 : Gain  Gain=-M(2,3)-Ma(2,3)  Multiplication=Matrix(K*u)  SaturateOnIntegerOverflow=on  OutDataTypeStr=Inherit: Same as input  ParamDataTypeStr=Inherit: Same as input
  Add : Sum
  Math Function : Math  Operator=magnitude^2  SignedPower=on  SaturateOnIntegerOverflow=on
  Product : Product  RndMeth=Zero
  x direction : Outport
  wires:
  v/1 -> Product/1
  r/1 -> Product/2, Math Function/1
  Product/1 -> -a22/1
  Math Function/1 -> -a26/1
  -a22/1 -> Add/1
  -a26/1 -> Add/2
  Add/1 -> x direction/1

== system towing_project/MotherShip/Coriolis and centripetal forces/Subsystem1 ==
  u : Inport
  r : Inport  Port=2
  Product : Product  RndMeth=Zero
  a11 : Gain  Gain=M(1,1)+Ma(1,1)  Multiplication=Matrix(K*u)  SaturateOnIntegerOverflow=on  OutDataTypeStr=Inherit: Same as input  ParamDataTypeStr=Inherit: Same as input
  y direction : Outport
  wires:
  Product/1 -> a11/1
  r/1 -> Product/2
  u/1 -> Product/1
  a11/1 -> y direction/1

== system towing_project/MotherShip/Coriolis and centripetal forces/Subsystem2 ==
  u : Inport
  v : Inport  Port=2
  r : Inport  Port=3
  Add : Sum
  Add1 : Sum  Inputs=+-
  Product : Product  RndMeth=Zero
  Product1 : Product  RndMeth=Zero
  a11 : Gain  Gain=M(1,1)+Ma(1,1)  Multiplication=Matrix(K*u)  SaturateOnIntegerOverflow=on  OutDataTypeStr=Inherit: Same as input  ParamDataTypeStr=Inherit: Same as input
  a22 : Gain  Gain=M(2,2)+Ma(2,2)  Multiplication=Matrix(K*u)  SaturateOnIntegerOverflow=on  OutDataTypeStr=Inherit: Same as input  ParamDataTypeStr=Inherit: Same as input
  a62 : Gain  Gain=M(3,2)+Ma(3,2)  Multiplication=Matrix(K*u)  SaturateOnIntegerOverflow=on  OutDataTypeStr=Inherit: Same as input  ParamDataTypeStr=Inherit: Same as input
  yaw direction : Outport
  wires:
  u/1 -> Product/1, Product1/1
  r/1 -> Product/2
  Product/1 -> a62/1
  v/1 -> Product1/2
  Product1/1 -> a22/1, a11/1
  a22/1 -> Add1/1
  a11/1 -> Add1/2
  Add1/1 -> Add/2
  a62/1 -> Add/1
  Add/1 -> yaw direction/1

== system towing_project/local DP1/Tug/Coriolis and centripetal forces ==
  nu : Inport
  Mux : Mux  Inputs=3
  Selector1 : Selector  InputPortWidth=3  IndexOptions=Index vector (dialog)  Indices=[1 ]  OutputSizes=1
  Selector2 : Selector  InputPortWidth=3  IndexOptions=Index vector (dialog)  Indices=[2]  OutputSizes=1
  Selector3 : Selector  InputPortWidth=3  IndexOptions=Index vector (dialog)  Indices=[3]  OutputSizes=1
  Subsystem : Subsystem
  Subsystem1 : Subsystem
  Subsystem2 : Subsystem
  Output : Outport
  wires:
  nu/1 -> Selector1/1, Selector2/1, Selector3/1
  Selector2/1 -> Subsystem/1(v), Subsystem2/2(v)  "v"
  Selector3/1 -> Subsystem/2(r), Subsystem1/2(r), Subsystem2/3(r)  "r"
  Selector1/1 -> Subsystem1/1(u), Subsystem2/1(u)  "u"
  Subsystem/1(x direction) -> Mux/1
  Subsystem1/1(y direction) -> Mux/2
  Subsystem2/1(yaw direction) -> Mux/3
  Mux/1 -> Output/1

== system towing_project/local DP1/Tug/In Case of singularity ==
  input : Inport
  Compare To Constant : simulink/Logic and Bit Operations/Compare To Constant  relop=>=  const=1e8  OutDataTypeStr=boolean
  Stop Simulation : Stop
  output : Outport
  wires:
  input/1 -> output/1, Compare To Constant/1
  Compare To Constant/1 -> Stop Simulation/1

== system towing_project/local DP1/Tug/In Case of singularity1 ==
  input : Inport
  Compare To Constant : simulink/Logic and Bit Operations/Compare To Constant  relop=>=  const=1e10  OutDataTypeStr=boolean
  Stop Simulation : Stop
  output : Outport
  wires:
  input/1 -> output/1, Compare To Constant/1
  Compare To Constant/1 -> Stop Simulation/1

== system towing_project/local DP1/Tug/Rotation matrix in yaw ==
  psi : Inport
  nu : Inport  Port=2
  Fcn : Fcn  Expr=cos(u(1))*u(2)-sin(u(1))*u(3)
  Fcn1 : Fcn  Expr=sin(u(1))*u(2)+cos(u(1))*u(3)
  Fcn2 : Fcn  Expr=u(4)
  Mux : Mux  Inputs=2
  Mux1 : Mux  Inputs=3
  R*nu : Outport
  wires:
  Mux1/1 -> R*nu/1  "eta_dot"
  Mux/1 -> Fcn/1, Fcn1/1, Fcn2/1
  psi/1 -> Mux/1
  nu/1 -> Mux/2
  Fcn1/1 -> Mux1/2  "y_dot"
  Fcn/1 -> Mux1/1  "x_dot"
  Fcn2/1 -> Mux1/3  "psi_dot"

== system towing_project/local DP1/Tug/[-inf inf] to [-pi pi]1 ==
  note: x
  note: r
  x [-inf inf] : Inport
  Constant : Constant  Value=2*pi
  Gain : Gain  Gain=pi  SaturateOnIntegerOverflow=on  OutDataTypeStr=Inherit: Same as input  ParamDataTypeStr=Inherit: Same as input
  Math Function : Math  Operator=rem  SignedPower=on  SaturateOnIntegerOverflow=on
  Saturation : Saturate  UpperLimit=1e10  LowerLimit=-1e10
  Sign : Signum
  Sum : Sum  Inputs=|+-  SaturateOnIntegerOverflow=on
  Sum1 : Sum  Inputs=|++  SaturateOnIntegerOverflow=on
  y [-pi pi] : Outport
  wires:
  x [-inf inf]/1 -> Saturation/1
  Sign/1 -> Gain/1
  Gain/1 -> Sum/2, Sum1/2
  Sum1/1 -> Math Function/1
  Constant/1 -> Math Function/2
  Math Function/1 -> Sum/1
  Sum/1 -> y [-pi pi]/1
  Saturation/1 -> Sum1/1, Sign/1

== system towing_project/local DP1/Tug DP controller/Transposed rotation  matrix in yaw ==
  psi : Inport
  V : Inport  Port=2
  Mux : Mux  Inputs=2
  Mux1 : Mux  Inputs=3
  Row1 : Fcn  Expr=cos(u(1))*u(2)+sin(u(1))*u(3)
  Row2 : Fcn  Expr=-sin(u(1))*u(2)+cos(u(1))*u(3)
  Row3 : Fcn  Expr=u(4)
  Out1 : Outport
  wires:
  Mux/1 -> Row3/1, Row2/1, Row1/1
  Row1/1 -> Mux1/1
  Row2/1 -> Mux1/2
  Row3/1 -> Mux1/3
  Mux1/1 -> Out1/1
  psi/1 -> Mux/1
  V/1 -> Mux/2

== system towing_project/local DP1/Tug DP controller/[-inf inf] to [-pi pi]1 ==
  note: x
  note: r
  x [-inf inf] : Inport
  Constant : Constant  Value=2*pi
  Gain : Gain  Gain=pi  SaturateOnIntegerOverflow=on  OutDataTypeStr=Inherit: Same as input  ParamDataTypeStr=Inherit: Same as input
  Math Function : Math  Operator=rem  SignedPower=on  SaturateOnIntegerOverflow=on
  Saturation : Saturate  UpperLimit=1e10  LowerLimit=-1e10
  Sign : Signum
  Sum : Sum  Inputs=|+-  SaturateOnIntegerOverflow=on
  Sum1 : Sum  Inputs=|++  SaturateOnIntegerOverflow=on
  y [-pi pi] : Outport
  wires:
  x [-inf inf]/1 -> Saturation/1
  Sign/1 -> Gain/1
  Gain/1 -> Sum/2, Sum1/2
  Sum1/1 -> Math Function/1
  Constant/1 -> Math Function/2
  Math Function/1 -> Sum/1
  Sum/1 -> y [-pi pi]/1
  Saturation/1 -> Sum1/1, Sign/1

== system towing_project/local DP1/Tug DP controller/[-inf inf] to [-pi pi]2 ==
  note: r
  note: x
  x [-inf inf] : Inport
  Constant : Constant  Value=2*pi
  Gain : Gain  Gain=pi  SaturateOnIntegerOverflow=on  OutDataTypeStr=Inherit: Same as input  ParamDataTypeStr=Inherit: Same as input
  Math Function : Math  Operator=rem  SignedPower=on  SaturateOnIntegerOverflow=on
  Saturation : Saturate  UpperLimit=1e10  LowerLimit=-1e10
  Sign : Signum
  Sum : Sum  Inputs=|+-  SaturateOnIntegerOverflow=on
  Sum1 : Sum  Inputs=|++  SaturateOnIntegerOverflow=on
  y [-pi pi] : Outport
  wires:
  Saturation/1 -> Sign/1, Sum1/1
  Sum/1 -> y [-pi pi]/1
  Math Function/1 -> Sum/1
  Constant/1 -> Math Function/2
  Sum1/1 -> Math Function/1
  Gain/1 -> Sum1/2, Sum/2
  Sign/1 -> Gain/1
  x [-inf inf]/1 -> Saturation/1

== system towing_project/local DP2/Tug/Coriolis and centripetal forces ==
  nu : Inport
  Mux : Mux  Inputs=3
  Selector1 : Selector  InputPortWidth=3  IndexOptions=Index vector (dialog)  Indices=[1 ]  OutputSizes=1
  Selector2 : Selector  InputPortWidth=3  IndexOptions=Index vector (dialog)  Indices=[2]  OutputSizes=1
  Selector3 : Selector  InputPortWidth=3  IndexOptions=Index vector (dialog)  Indices=[3]  OutputSizes=1
  Subsystem : Subsystem
  Subsystem1 : Subsystem
  Subsystem2 : Subsystem
  Output : Outport
  wires:
  nu/1 -> Selector1/1, Selector2/1, Selector3/1
  Selector2/1 -> Subsystem/1(v), Subsystem2/2(v)  "v"
  Selector3/1 -> Subsystem/2(r), Subsystem1/2(r), Subsystem2/3(r)  "r"
  Selector1/1 -> Subsystem1/1(u), Subsystem2/1(u)  "u"
  Subsystem/1(x direction) -> Mux/1
  Subsystem1/1(y direction) -> Mux/2
  Subsystem2/1(yaw direction) -> Mux/3
  Mux/1 -> Output/1

== system towing_project/local DP2/Tug/In Case of singularity ==
  input : Inport
  Compare To Constant : simulink/Logic and Bit Operations/Compare To Constant  relop=>=  const=1e8  OutDataTypeStr=boolean
  Stop Simulation : Stop
  output : Outport
  wires:
  input/1 -> output/1, Compare To Constant/1
  Compare To Constant/1 -> Stop Simulation/1

== system towing_project/local DP2/Tug/In Case of singularity1 ==
  input : Inport
  Compare To Constant : simulink/Logic and Bit Operations/Compare To Constant  relop=>=  const=1e10  OutDataTypeStr=boolean
  Stop Simulation : Stop
  output : Outport
  wires:
  input/1 -> output/1, Compare To Constant/1
  Compare To Constant/1 -> Stop Simulation/1

== system towing_project/local DP2/Tug/Rotation matrix in yaw ==
  psi : Inport
  nu : Inport  Port=2
  Fcn : Fcn  Expr=cos(u(1))*u(2)-sin(u(1))*u(3)
  Fcn1 : Fcn  Expr=sin(u(1))*u(2)+cos(u(1))*u(3)
  Fcn2 : Fcn  Expr=u(4)
  Mux : Mux  Inputs=2
  Mux1 : Mux  Inputs=3
  R*nu : Outport
  wires:
  Mux1/1 -> R*nu/1  "eta_dot"
  Mux/1 -> Fcn/1, Fcn1/1, Fcn2/1
  psi/1 -> Mux/1
  nu/1 -> Mux/2
  Fcn1/1 -> Mux1/2  "y_dot"
  Fcn/1 -> Mux1/1  "x_dot"
  Fcn2/1 -> Mux1/3  "psi_dot"

== system towing_project/local DP2/Tug/[-inf inf] to [-pi pi]1 ==
  note: x
  note: r
  x [-inf inf] : Inport
  Constant : Constant  Value=2*pi
  Gain : Gain  Gain=pi  SaturateOnIntegerOverflow=on  OutDataTypeStr=Inherit: Same as input  ParamDataTypeStr=Inherit: Same as input
  Math Function : Math  Operator=rem  SignedPower=on  SaturateOnIntegerOverflow=on
  Saturation : Saturate  UpperLimit=1e10  LowerLimit=-1e10
  Sign : Signum
  Sum : Sum  Inputs=|+-  SaturateOnIntegerOverflow=on
  Sum1 : Sum  Inputs=|++  SaturateOnIntegerOverflow=on
  y [-pi pi] : Outport
  wires:
  x [-inf inf]/1 -> Saturation/1
  Sign/1 -> Gain/1
  Gain/1 -> Sum/2, Sum1/2
  Sum1/1 -> Math Function/1
  Constant/1 -> Math Function/2
  Math Function/1 -> Sum/1
  Sum/1 -> y [-pi pi]/1
  Saturation/1 -> Sum1/1, Sign/1

== system towing_project/local DP2/Tug DP controller/Transposed rotation  matrix in yaw ==
  psi : Inport
  V : Inport  Port=2
  Mux : Mux  Inputs=2
  Mux1 : Mux  Inputs=3
  Row1 : Fcn  Expr=cos(u(1))*u(2)+sin(u(1))*u(3)
  Row2 : Fcn  Expr=-sin(u(1))*u(2)+cos(u(1))*u(3)
  Row3 : Fcn  Expr=u(4)
  Out1 : Outport
  wires:
  Mux/1 -> Row3/1, Row2/1, Row1/1
  Row1/1 -> Mux1/1
  Row2/1 -> Mux1/2
  Row3/1 -> Mux1/3
  Mux1/1 -> Out1/1
  psi/1 -> Mux/1
  V/1 -> Mux/2

== system towing_project/local DP2/Tug DP controller/[-inf inf] to [-pi pi]1 ==
  note: x
  note: r
  x [-inf inf] : Inport
  Constant : Constant  Value=2*pi
  Gain : Gain  Gain=pi  SaturateOnIntegerOverflow=on  OutDataTypeStr=Inherit: Same as input  ParamDataTypeStr=Inherit: Same as input
  Math Function : Math  Operator=rem  SignedPower=on  SaturateOnIntegerOverflow=on
  Saturation : Saturate  UpperLimit=1e10  LowerLimit=-1e10
  Sign : Signum
  Sum : Sum  Inputs=|+-  SaturateOnIntegerOverflow=on
  Sum1 : Sum  Inputs=|++  SaturateOnIntegerOverflow=on
  y [-pi pi] : Outport
  wires:
  x [-inf inf]/1 -> Saturation/1
  Sign/1 -> Gain/1
  Gain/1 -> Sum/2, Sum1/2
  Sum1/1 -> Math Function/1
  Constant/1 -> Math Function/2
  Math Function/1 -> Sum/1
  Sum/1 -> y [-pi pi]/1
  Saturation/1 -> Sum1/1, Sign/1

== system towing_project/local DP2/Tug DP controller/[-inf inf] to [-pi pi]2 ==
  note: r
  note: x
  x [-inf inf] : Inport
  Constant : Constant  Value=2*pi
  Gain : Gain  Gain=pi  SaturateOnIntegerOverflow=on  OutDataTypeStr=Inherit: Same as input  ParamDataTypeStr=Inherit: Same as input
  Math Function : Math  Operator=rem  SignedPower=on  SaturateOnIntegerOverflow=on
  Saturation : Saturate  UpperLimit=1e10  LowerLimit=-1e10
  Sign : Signum
  Sum : Sum  Inputs=|+-  SaturateOnIntegerOverflow=on
  Sum1 : Sum  Inputs=|++  SaturateOnIntegerOverflow=on
  y [-pi pi] : Outport
  wires:
  Saturation/1 -> Sign/1, Sum1/1
  Sum/1 -> y [-pi pi]/1
  Math Function/1 -> Sum/1
  Constant/1 -> Math Function/2
  Sum1/1 -> Math Function/1
  Gain/1 -> Sum1/2, Sum/2
  Sign/1 -> Gain/1
  x [-inf inf]/1 -> Saturation/1

== system towing_project/local DP1/Tug/Coriolis and centripetal forces/Subsystem ==
  v : Inport
  r : Inport  Port=2
  -a22 : Gain  Gain=-M1(2,2)-Ma1(2,2)  Multiplication=Matrix(K*u)  SaturateOnIntegerOverflow=on  OutDataTypeStr=Inherit: Same as input  ParamDataTypeStr=Inherit: Same as input
  -a26 : Gain  Gain=-M1(2,3)-Ma1(2,3)  Multiplication=Matrix(K*u)  SaturateOnIntegerOverflow=on  OutDataTypeStr=Inherit: Same as input  ParamDataTypeStr=Inherit: Same as input
  Add : Sum
  Math Function : Math  Operator=magnitude^2  SignedPower=on  SaturateOnIntegerOverflow=on
  Product : Product  RndMeth=Zero
  x direction : Outport
  wires:
  v/1 -> Product/1
  r/1 -> Product/2, Math Function/1
  Product/1 -> -a22/1
  Math Function/1 -> -a26/1
  -a22/1 -> Add/1
  -a26/1 -> Add/2
  Add/1 -> x direction/1

== system towing_project/local DP1/Tug/Coriolis and centripetal forces/Subsystem1 ==
  u : Inport
  r : Inport  Port=2
  Product : Product  RndMeth=Zero
  a11 : Gain  Gain=M1(1,1)+Ma1(1,1)  Multiplication=Matrix(K*u)  SaturateOnIntegerOverflow=on  OutDataTypeStr=Inherit: Same as input  ParamDataTypeStr=Inherit: Same as input
  y direction : Outport
  wires:
  Product/1 -> a11/1
  r/1 -> Product/2
  u/1 -> Product/1
  a11/1 -> y direction/1

== system towing_project/local DP1/Tug/Coriolis and centripetal forces/Subsystem2 ==
  u : Inport
  v : Inport  Port=2
  r : Inport  Port=3
  Add : Sum
  Add1 : Sum  Inputs=+-
  Product : Product  RndMeth=Zero
  Product1 : Product  RndMeth=Zero
  a11 : Gain  Gain=M1(1,1)+Ma1(1,1)  Multiplication=Matrix(K*u)  SaturateOnIntegerOverflow=on  OutDataTypeStr=Inherit: Same as input  ParamDataTypeStr=Inherit: Same as input
  a22 : Gain  Gain=M1(2,2)+Ma1(2,2)  Multiplication=Matrix(K*u)  SaturateOnIntegerOverflow=on  OutDataTypeStr=Inherit: Same as input  ParamDataTypeStr=Inherit: Same as input
  a62 : Gain  Gain=M1(3,2)+Ma1(3,2)  Multiplication=Matrix(K*u)  SaturateOnIntegerOverflow=on  OutDataTypeStr=Inherit: Same as input  ParamDataTypeStr=Inherit: Same as input
  yaw direction : Outport
  wires:
  u/1 -> Product/1, Product1/1
  r/1 -> Product/2
  Product/1 -> a62/1
  v/1 -> Product1/2
  Product1/1 -> a22/1, a11/1
  a22/1 -> Add1/1
  a11/1 -> Add1/2
  Add1/1 -> Add/2
  a62/1 -> Add/1
  Add/1 -> yaw direction/1

== system towing_project/local DP2/Tug/Coriolis and centripetal forces/Subsystem ==
  v : Inport
  r : Inport  Port=2
  -a22 : Gain  Gain=-M1(2,2)-Ma1(2,2)  Multiplication=Matrix(K*u)  SaturateOnIntegerOverflow=on  OutDataTypeStr=Inherit: Same as input  ParamDataTypeStr=Inherit: Same as input
  -a26 : Gain  Gain=-M1(2,3)-Ma1(2,3)  Multiplication=Matrix(K*u)  SaturateOnIntegerOverflow=on  OutDataTypeStr=Inherit: Same as input  ParamDataTypeStr=Inherit: Same as input
  Add : Sum
  Math Function : Math  Operator=magnitude^2  SignedPower=on  SaturateOnIntegerOverflow=on
  Product : Product  RndMeth=Zero
  x direction : Outport
  wires:
  v/1 -> Product/1
  r/1 -> Product/2, Math Function/1
  Product/1 -> -a22/1
  Math Function/1 -> -a26/1
  -a22/1 -> Add/1
  -a26/1 -> Add/2
  Add/1 -> x direction/1

== system towing_project/local DP2/Tug/Coriolis and centripetal forces/Subsystem1 ==
  u : Inport
  r : Inport  Port=2
  Product : Product  RndMeth=Zero
  a11 : Gain  Gain=M1(1,1)+Ma1(1,1)  Multiplication=Matrix(K*u)  SaturateOnIntegerOverflow=on  OutDataTypeStr=Inherit: Same as input  ParamDataTypeStr=Inherit: Same as input
  y direction : Outport
  wires:
  Product/1 -> a11/1
  r/1 -> Product/2
  u/1 -> Product/1
  a11/1 -> y direction/1

== system towing_project/local DP2/Tug/Coriolis and centripetal forces/Subsystem2 ==
  u : Inport
  v : Inport  Port=2
  r : Inport  Port=3
  Add : Sum
  Add1 : Sum  Inputs=+-
  Product : Product  RndMeth=Zero
  Product1 : Product  RndMeth=Zero
  a11 : Gain  Gain=M1(1,1)+Ma1(1,1)  Multiplication=Matrix(K*u)  SaturateOnIntegerOverflow=on  OutDataTypeStr=Inherit: Same as input  ParamDataTypeStr=Inherit: Same as input
  a22 : Gain  Gain=M1(2,2)+Ma1(2,2)  Multiplication=Matrix(K*u)  SaturateOnIntegerOverflow=on  OutDataTypeStr=Inherit: Same as input  ParamDataTypeStr=Inherit: Same as input
  a62 : Gain  Gain=M1(3,2)+Ma1(3,2)  Multiplication=Matrix(K*u)  SaturateOnIntegerOverflow=on  OutDataTypeStr=Inherit: Same as input  ParamDataTypeStr=Inherit: Same as input
  yaw direction : Outport
  wires:
  u/1 -> Product/1, Product1/1
  r/1 -> Product/2
  Product/1 -> a62/1
  v/1 -> Product1/2
  Product1/1 -> a22/1, a11/1
  a22/1 -> Add1/1
  a11/1 -> Add1/2
  Add1/1 -> Add/2
  a62/1 -> Add/1
  Add/1 -> yaw direction/1

== matlab function Cable Force ==
  data: state input double; tau1 output double; tau2 output double
function [tau1, tau2] = cable_force(state)

%% 锚链
    Kc = 6e4;
    L10 = 400;
    L20 = 400;
    
    x0 = [-75, 75, 75, -75, -75];
    y0 = [50, 50, -50, -50, 50];
    x1 = [-16, 12, 16, 12, -16, -16];
    y1 = [6, 6, 0, -6, -6, 6];
    x2 = [-16, 12, 16, 12, -16, -16];
    y2 = [6, 6, 0, -6, -6, 6];
    
    p0 = state(1 : 3);
    p1 = state(7 : 9);
    p2 = state(13 : 15);
    
    % 角度转化成弧度
    p0(3) = p0(3) * pi / 180;
    p1(3) = p1(3) * pi / 180;
    p2(3) = p2(3) * pi / 180;
    
    % 缆绳起始点坐标（全局坐标系下）
    pc1_start = local_to_global([x0(2); y0(2)], p0);
    pc1_end = local_to_global([(x1(1)+x1(5))/2; (y1(1)+y1(5))/2], p1);
    pc2_start = local_to_global([x0(3); y0(3)], p0);
    pc2_end = local_to_global([(x2(1)+x2(5))/2; (y2(1)+y2(5))/2], p2);
    
    
    % 缆绳长度
    Lc1 = sqrt((pc1_start(1) - pc1_end(1)) ^ 2 + (pc1_start(2) - pc1_end(2)) ^ 2 );
    Lc2 = sqrt((pc2_start(1) - pc2_end(1)) ^ 2 + (pc2_start(2) - pc2_end(2)) ^ 2 );
    
    % 缆绳张力
    fc1 = Kc * (Lc1 - L10);
    fc2 = Kc * (Lc2 - L20);
    
    
    % 缆绳角度
    alpha1 = atan2( -(pc1_start(2) - pc1_end(2)), -(pc1_start(1) - pc1_end(1)) );
    alpha2 = atan2( -(pc2_start(2) - pc2_end(2)), -(pc2_start(1) - pc2_end(1)) );
    
    % 缆绳相对母船的角度（母船坐标系下）
    belta1 = alpha1 - p0(3);
    belta2 = alpha2 - p0(3);
    
    % 将角度转化为（-pi, pi)
    belta1 = transfer_deg(belta1);
    belta2 = transfer_deg(belta2);
    
    tau1 = fc1 * [ cos(belta1),  sin(belta1), y0(2) * sin(belta1) - x0(2) * cos(belta1) ]';
    tau2 = fc2 * [ cos(belta2),  sin(belta2), y0(3) * sin(belta2) - x0(3) * cos(belta2) ]';
end


%% 寻找锚链连接点(大地坐标系下）
function pc_g = local_to_global(pc_l, p0)
    fai = p0(3);
    R = [cos(fai), -sin(fai);
        sin(fai), cos(fai)];
    pc_g = R * pc_l + p0(1:2);
    
end

%% 旋转矩阵
function [R2, R3] = rotate_matrix(p)

    fai = p(3);
    R2  = [cos(fai), -sin(fai);
            sin(fai), cos(fai)];
    
    R3 = [cos(fai), -sin(fai), 0;
        sin(fai), cos(fai), 0;
        0, 0, 1];
end

%% 将角度转化为（-pi, pi)
function y = transfer_deg(x)
    y = -sign(x) * pi + rem((x + sign(x) * pi), 2 * pi);
end

== matlab function Consensus Control ==
  data: p0 input double; pd1 output double; v0 input double; state input double; pd2 output double
% function [pd1, pd2] = consensus_guidance(p0, v0, p1, v1, p2, v2)
function [pd1, pd2] = consensus_guidance(p0, v0, state)
% 默认输入和输出的单位为角度
% % p0, v0的角度单位都是弧度
% p(全局坐标系）， v(局部坐标系）
% dot_p (全局坐标系）
% clear all; clc;
% p1 = [397, 237, 31]';
% p2 = [397, -237, -31]';
% p0 = [1, 0, 0]';
% v0 = zeros(3, 1);
% v1 = zeros(3, 1);
% v2 = zeros(3, 1);

p1 = state(1:3);
v1 = state(4:6);
p2 = state(7:9);
v2 = state(10:12);

% 需要声明lqr函数为外部函数，否则simulink会编译报错
coder.extrinsic('lqr'); 

pd1 = zeros(3, 1);
pd2 = zeros(3, 1);

% 角度单位转化成弧度
deg_to_rad = pi / 180;
p0(3) = p0(3) * deg_to_rad;
p1(3) = p1(3) * deg_to_rad;
p2(3) = p2(3) * deg_to_rad;
dotP0 = v0;     
dotP0(3) = dotP0(3) * deg_to_rad;

% % 将角度转化为（-pi, pi)
p0(3) = transfer_deg(p0(3));
p1(3) = transfer_deg(p1(3));
p2(3) = transfer_deg(p2(3));

% dotP0 = V_to_dotP(p0, v0);
dotP1 = V_to_dotP(p1, v1);
dotP2 = V_to_dotP(p2, v2);
% 定义状态变量
x0 = [p0; dotP0];
x1 = [p1; dotP1];
x2 = [p2; dotP2];

%% 编队的相对位置,这个是在局部坐标系下的，需要转化为大地坐标系下
deta10 = [397, 237, 31 * deg_to_rad, 0, 0, 0]';
deta20 = [397, -237, -31 * deg_to_rad, 0, 0, 0]';
deta12 = [0, 474, 62 * deg_to_rad, 0, 0, 0]';
deta21 = -[0, 474, 62 * deg_to_rad, 0, 0, 0]';
fai0 = p0(3);   fai1 = p1(3);   fai2 = p2(3);
Lc1 = sqrt(deta10(1)^2 + deta10(2)^2);
Lc2 = sqrt(deta20(1)^2 + deta20(2)^2);

deta10(1:2) = [cos(fai0), -sin(fai0); sin(fai0), cos(fai0)] * deta10(1:2);
deta20(1:2) = [cos(fai0), -sin(fai0); sin(fai0), cos(fai0)] * deta20(1:2);

deta12 = deta10 - deta20;
deta21 = - deta12;



% 先假定aij = 1, gi = 1;， 需要加上相对位置
e1 = x2 - x1 - deta21 + x0 - x1 + deta10;
e2 = x1 - x2 - deta12 + x0 - x2 + deta20;

% % 将角度误差转化为（-pi, pi),这个很重要
e1(3) = transfer_deg(e1(3));
e2(3) = transfer_deg(e2(3));

%% 定义状态反馈方程的系数，求解raccati方程
wn = 0.05; 
cd = 0.7;

A1 = -2 * cd * wn * eye(3);
A0 = -wn^2 * eye(3);
B1 = -A0;

A = [zeros(3, 3), eye(3); A0, A1];
B = [zeros(3, 3); B1];

% Q = diag([0.01, 0.01, 4e-8, 100, 100, 4e-4]);
% R = diag([0.01, 0.01, 4e-8]);
Q = 4 * eye(6);
R = 1 * eye(3);
N = [];
[K, S, e] = lqr(A, B, Q, R, N);

K;
u1 = K * e1;
u2 = K * e2;

pd1 = u1; 
pd2 = u2;

pd1 = pd1 + p1;
pd2 = pd2 + p2;
pd1(3) = transfer_deg(pd1(3));
pd2(3) = transfer_deg(pd2(3));


%% 函数输入输出都是角度
pd1(3) = pd1(3) / 3.14 * 180;
pd2(3) = pd2(3) / 3.14 * 180;

end







%% 旋转矩阵
function R = RotationMatrix(p)
fai = p(3);
R = zeros(3, 3);
R = [cos(fai), -sin(fai), 0;
    sin(fai), cos(fai), 0;
    0, 0, 1];
end

%% 将速度转换成全局坐标系中，即p的微分
function dot_P = V_to_dotP(p, v)
R = zeros(3, 3);
R = RotationMatrix(p);
dot_P = R * v;

end

%% 将角度转化为（-pi, pi)
function y = transfer_deg(x)
    y = -sign(x) * pi + rem((x + sign(x) * pi), 2 * pi);
end
